simulink model "Lezione7model"  (R2022b)
settings: Solver=VariableStepAuto  StartTime=0.0  StopTime=30.0  RelTol=1e-3
libraries: cstblocks x4
settings Model: Creator=giov_russo  LastModifiedBy=Ares-

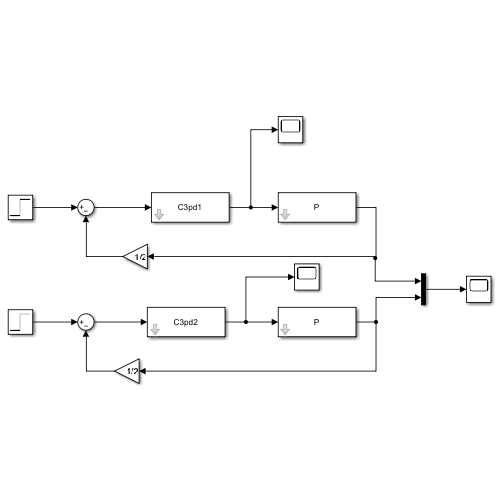
[thumbnail: Simulink's stored preview of the top-level diagram]
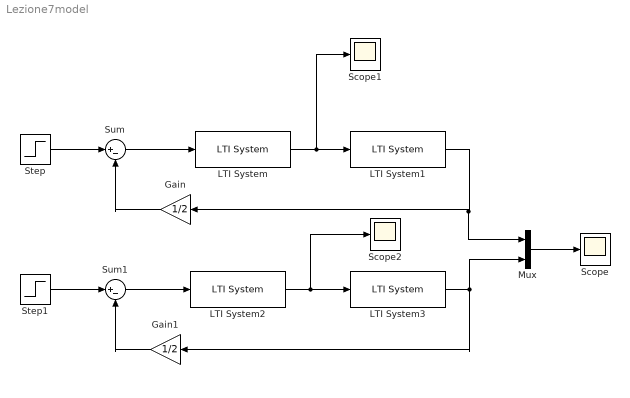
== system Lezione7model ==
  Gain : Gain  Gain=1/2
  Gain1 : Gain  Gain=1/2
  LTI System : cstblocks/LTI System  sys=C3pd1  IC=[]
  LTI System1 : cstblocks/LTI System  sys=P  IC=[]
  LTI System2 : cstblocks/LTI System  sys=C3pd2  IC=[]
  LTI System3 : cstblocks/LTI System  sys=P  IC=[]
  Mux : Mux  Inputs=2
  Scope : Scope
  Scope1 : Scope
  Scope2 : Scope
  Step : Step  Time=0  SampleTime=0
  Step1 : Step  Time=0  SampleTime=0
  Sum : Sum  Inputs=|+-
  Sum1 : Sum  Inputs=|+-
  wires:
  LTI System/1 -> Scope1/1, LTI System1/1
  Sum/1 -> LTI System/1
  LTI System1/1 -> Mux/1, Gain/1
  Step/1 -> Sum/1
  Sum1/1 -> LTI System2/1
  LTI System3/1 -> Mux/2, Gain1/1
  LTI System2/1 -> Scope2/1, LTI System3/1
  Step1/1 -> Sum1/1
  Mux/1 -> Scope/1
  Gain/1 -> Sum/2
  Gain1/1 -> Sum1/2
